simulink model "Place3"  (R2019a)
settings: Solver=VariableStepAuto  StartTime=0.0  StopTime=10.0  RelTol=1e-3
settings Model: Creator=anton  LastModifiedBy=anton

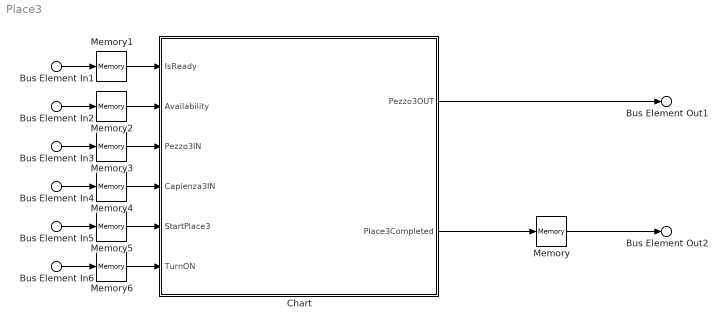
== system Place3 ==
  Bus Element In1 : Inport  PortName=IsReady
  Bus Element In3 : Inport  Port=2  PortName=Pezzo3IN
  Bus Element In4 : Inport  Port=3  PortName=Capienza3IN
  Bus Element In5 : Inport  Port=4  PortName=StartPlace3
  Bus Element In6 : Inport  Port=5  PortName=TurnON
  Bus Element In2 : Inport  Port=6  PortName=AvailabilityIN
  Chart : Stateflow chart  BlockKeywords=__PRM__SERIALIZED__DATA__:Stateflow Chart,Stateflow Diagram  TreatAsAtomicUnit=on
  Memory{,1..6} (7 alike) : Memory
  Bus Element Out1 : Outport  PortName=Pezzo3OUT
  Bus Element Out2 : Outport  Port=2  PortName=Place3Completed
  wires:
  Chart/1(Pezzo3OUT) -> Bus Element Out1/1
  Chart/2(Place3Completed) -> Memory/1
  Memory/1 -> Bus Element Out2/1
  Bus Element In6/1 -> Memory6/1
  Memory6/1 -> Chart/6(TurnON)
  Bus Element In5/1 -> Memory5/1
  Memory5/1 -> Chart/5(StartPlace3)
  Bus Element In4/1 -> Memory4/1
  Memory4/1 -> Chart/4(Capienza3IN)
  Bus Element In3/1 -> Memory3/1
  Memory3/1 -> Chart/3(Pezzo3IN)
  Bus Element In2/1 -> Memory2/1
  Memory2/1 -> Chart/2(Availability)
  Bus Element In1/1 -> Memory1/1
  Memory1/1 -> Chart/1(IsReady)

== stateflow chart Place3/Chart ==
  state Idle
    Pezzo3OUT=0;
    Place3Completed=0;
  state Waiting
    Pezzo3OUT=0;
    Place3Completed=0;
  state Active1
  state Working
  state Place
    during:
    Pezzo3OUT=1;
    Place3Completed = 1;
    pause(0.1);
  state Pick
    pause(0.1);
  (default) -> Idle
  Idle -> Active1 : [TurnON==1]
  Place -> Idle [order 2] : [TurnON==0]
  Waiting -> Idle [order 2] : [TurnON==0]
  Pick -> Idle [order 2] : [TurnON==0]
  Working -> Idle [order 2] : [TurnON==0]
  Active1 -> Waiting
  Waiting -> Working [order 1] : [StartPlace3==1]
  Place -> Waiting [order 1] : [after(1,sec)]
  Working -> Pick [order 1] : [IsReady==1 && Availability==1 && Pezzo3IN==1 && Capienza3IN<6]
  Pick -> Place [order 1] : [after(10,sec)]
  data: IsReady input; Availability input; Pezzo3IN input; Capienza3IN input; StartPlace3 input; Pezzo3OUT output; Place3Completed output; TurnON input
